simulink library "stopwatch_ul"  (R2022a)
settings: Solver=VariableStepAuto  StartTime=0.0  StopTime=10.0  RelTol=1e-3
settings Model: Creator=mcobb  LastModifiedBy=adabney
settings SolverCC: AlgebraicLoopSolver=TrustRegion
settings DebuggingCC: UnconnectedInputMsg=warning  UnconnectedOutputMsg=warning  UnconnectedLineMsg=warning  SFMachineParentedDataDiag=warning  ArithmeticOperatorsInVariantConditions=warning
settings SFSimCC: CustomCodeUndefinedFunction=UseInterfaceOnly

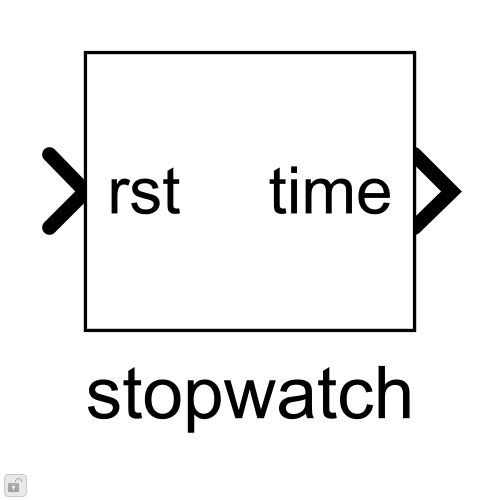
[thumbnail: Simulink's stored preview of the top-level diagram]
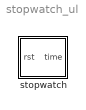
== system stopwatch_ul ==
  stopwatch : Subsystem

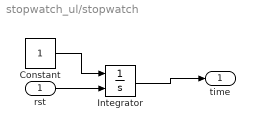
== system stopwatch_ul/stopwatch ==
  rst : Inport
  Constant : Constant
  Integrator : Integrator  ExternalReset=rising
  time : Outport  VectorParamsAs1DForOutWhenUnconnected=off
  wires:
  rst/1 -> Integrator/2
  Integrator/1 -> time/1
  Constant/1 -> Integrator/1
